simulink library "xblocks_library_pfbs"  (Simulink 7.6)
settings: Solver=ode45  SolverMode=SingleTasking  StartTime=0.0  StopTime=10.0  RelTol=1e-3
libraries: xbsIndex_r4 x369, monroe_library x47
(part 1 of 7)
settings Model: Creator=mdexter  LastModifiedBy=ptcs

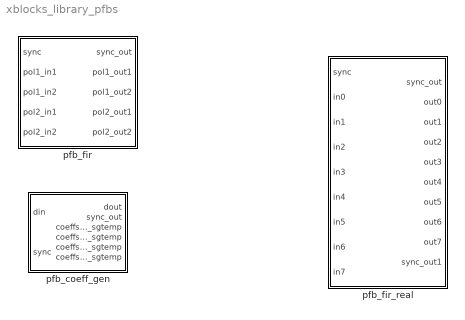
== system xblocks_library_pfbs ==
  pfb_coeff_gen : Subsystem  mask(pfb_coeff_gen){PFBSize=6, CoeffBitWidth=8, TotalTaps=4, CoeffDistMem=0, WindowType=hamming, bram_latency=2, n_inputs=0, nput=0, fwidth=1}
      mask prompts: PFBSize "Size of PFB: (2^? pnts)"; CoeffBitWidth "Bitwidth of Coefficients:"; TotalTaps "Total Number of Taps:"; CoeffDistMem "Implement Coeff Gen in Distributed Memory"; WindowType "Windowing Function:"; bram_latency "BRAM Latency"; n_inputs "Number of Simultaneous Inputs: (2^?)"; nput "This is input number:"; fwidth "Bin Width (normal=1)"
      mask init:
      | config.source = str2func('pfb_coeff_gen_init_xblock');
      | config.toplevel = gcb;
      | config.depend = get_dependlist('pfb_coeff_gen');
      | set_param(gcb,'LinkStatus','inactive');
      | xBlock(config, {config.toplevel, ...
      |     PFBSize, ...
      |     CoeffBitWidth, ...
      |     TotalTaps, ...
      |     CoeffDistMem, ...
      |     WindowType, ...
      |     bram_latency, ...
      |     n_inputs, ...
      |     nput, ...
      |     fwidth});
      settings: AttributesFormatString=PFBSize=6, n_inputs=0, taps=4
  pfb_fir : Subsystem  mask(pfb_fir){PFBSize=5, TotalTaps=2, WindowType=hamming, n_inputs=1, MakeBiplex=on, BitWidthIn=8, BitWidthOut=18, CoeffBitWidth=18, CoeffDistMem=off, add_latency=1, mult_latency=2, bram_latency=2, quantization=Round  (unbiased: +/- Inf), fwidth=1, oversample_factor=1, oversample_index=0, specify_mult=off, mult_spec=[2                                      2]}
      mask prompts: PFBSize "Size of PFB: (2^? pnts)"; TotalTaps "Total Number of Taps:"; WindowType "Windowing Function:"; n_inputs "Number of Simultaneous Inputs: (2^?)"; MakeBiplex "Make Biplex"; BitWidthIn "Input Bitwidth:"; BitWidthOut "Output Bitwidth:"; CoeffBitWidth "Coefficient Bitwidth:"; CoeffDistMem "Use Distributed Memory for Coeffs"; add_latency "Add Latency"; mult_latency "Mult Latency"; bram_latency "BRAM Latency"; quantization "Quantization Behavior"; fwidth "Bin Width Scaling (normal=1)"; oversample_factor "Oversampling factor"; oversample_index "Oversampling index"; specify_mult "Specify multiplier use (behavioral if not specified)"; mult_spec "Multiplier specification (0=core, 1=embedded, 2=behavioural) (left=1st tap)"
      mask init:
      | config.source = str2func('pfb_fir_init_xblock');
      | config.toplevel = gcb;
      | config.depend = get_dependlist('pfb_fir');
      | set_param(gcb,'LinkStatus','inactive');
      | xBlock(config,{config.toplevel, ...
      |     'PFBSize', PFBSize, ...
      |     'TotalTaps', TotalTaps, ...
      |     'WindowType', WindowType, ...
      |     'n_inputs', n_inputs, ...
      |     'MakeBiplex', MakeBiplex, ...
      |     'BitWidthIn', BitWidthIn, ...
      |     'BitWidthOut', BitWidthOut, ...
      |     'CoeffBitWidth', CoeffBitWidth, ...
      |     'CoeffDistMem', CoeffDistMem, ...
      |     'add_latency', add_latency, ...
      |     'mult_latency', mult_latency, ...
      |     'bram_latency', bram_latency, ...
      |     'quantization', quantization, ...
      |     'fwidth', fwidth,...
      |     'oversample_factor', oversample_factor,...
      |     'oversample_index', oversample_index,...
      |     'specify_mult', specify_mult,...
      |     'mult_spec', mult_spec});
      settings: AttributesFormatString=taps=2, add_latency=1
      mask Help: eval('xlWeb(''http://casper.berkeley.edu/wiki/Pfb_fir'')')
      mask StyleString: edit,edit,popup(bartlett|barthannwin|blackman|blackmanharris|bohamwin|chebwin|flattopwin|gausswin|hamming|hann|kaiser|nuttallwin|parzenwin|rectwin|tukeywin|triang|userwindow),edit,checkbox,edit,edit,edit,checkbox,edit,edit,edit,popup(Truncate|Round  (unbiased: +/- Inf)|Round  (unbiased: Even Values)),edit,edit,edit,checkbox,edit
      mask CallbackString:
      | |%num_taps = eval(get_param(gcb, 'TotalTaps'));
      | %old_vec = eval(get_param(gcb, 'mult_spec'));
      | 
      | %vec = 2.*ones(1,num_taps);
      | %old_size = length(old_vec);
      | 
      | %if(old_size <= num_taps),
      | %   new_size = old_size;
      | %else,
      | %    new_size = num_taps;
      | %end
      | 
      | %for n = 1:new_size, vec(n) = old_vec(n); end
      | %set_param(gcb, 'mult_spec', mat2str(vec));||||||||||||%num_taps = eval(get_param(gcb, 'TotalTaps'));
      | %old_vec = eval(get_param(gcb, 'mult_spec'));
      | 
      | %vec = 2.*ones(1,num_taps);
      | %old_size = length(old_vec);
      | 
      | %if(old_size <= num_taps),
      | %    new_size = old_size;
      | %else,
      | %    new_size = num_taps;
      | %end
      | 
      | %for n = 1:new_size, vec(n) = old_vec(n); end
      | %set_param(gcb, 'mult_spec', mat2str(vec));|||%specify_mult = get_param(gcb,'specify_mult');
      | %if( strcmp(specify_mult,'off')),
      | %    set_param(gcb, 'MaskEnables', {'on','on','on','on','on','on','on','on','on','on','on','on','on','on','on','off'});
      | %else
      | %    set_param(gcb, 'MaskEnables', {'on','on','on','on','on','on','on','on','on','on','on','on','on','on','on','on'});
      | %end
      | 
      | |%specify_mult = get_param(gcb,'specify_mult');
      | %if( strcmp(specify_mult,'off')),
      | %    set_param(gcb, 'MaskEnables', {'on','on','on','on','on','on','on','on','on','on','on','on','on','on','on','off'});
      | %else
      | %    set_param(gcb, 'MaskEnables', {'on','on','on','on','on','on','on','on','on','on','on','on','on','on','on','on'});
      | %end
  pfb_fir_real : Subsystem  mask(pfb_coeff_gen_dual){pfb_size=14, n_sim_inputs=3, n_taps=4, data_n_bits=18, coeff_n_bits=18, output_bit_width=18, window_fn=hamming, bin_width=1, end_scale_val=1, endDelay=off, cheap_sync=off, autoplace_mode='Attached to ADC0', autoplace_optimize=off, bram_latency_coeff=off, bram_latency_delay=off, register_counter=off, pack_delays=on}
      mask prompts: pfb_size "PFB Size (2^?)"; n_sim_inputs "# Simultaneous Inputs (2^?); Max=6"; n_taps "# Taps"; data_n_bits "Input bit Width"; coeff_n_bits "# Coefficient Bits"; output_bit_width "Output bit width"; window_fn "Window Function"; bin_width "Channel Width"; end_scale_val "Downscale at end (2^?)"; endDelay "Delay at end?"; cheap_sync "Use cheap Sync hardware?"; autoplace_mode "Autoplacement Mode?"; autoplace_optimize "Optimize parameters for auto-placement? (settings below here ignored)"; bram_latency_coeff "Register Coefficient Brams?"; bram_latency_delay "Register Delay Brams?"; register_counter "Register Delay Counters? (0 or 1)"; pack_delays "Pack delays cross-input?"
      mask init:
      | global drawing_parameters;
      | % drawing_parameters.pfb_size=pfb_size;
      | % drawing_parameters.n_sim_inputs=n_sim_inputs;
      | % drawing_parameters.n_taps=n_taps;
      | % drawing_parameters.data_n_bits=data_n_bits;
      | % drawing_parameters.data_bin_pt=data_bin_pt;
      | % drawing_parameters.coeff_n_bits=coeff_n_bits;
      | % drawing_parameters.coeff_bin_pt=coeff_n_bits-1;
      | % drawing_parameters.window_fn=window_fn;
      | % drawing_parameters.mem_type=mem_type;
      | % drawing_parameters.bram_latency=bram_latency;
      | % drawing_parameters.bin_width=bin_width;
      | % drawing_parameters.end_scale_val=end_scale_val;
      | % drawing_parameters.cheap_sync=cheap_sync;
      | config.source=str2func('pfb_improved_draw');
      | config.toplevel=gcb;
      | config.debug=0;
      | config.depend={'pfb_improved_draw.m','pfb_coeff_gen_dual_draw.m'};
      | xBlock(config,{pfb_size,n_sim_inputs,n_taps,data_n_bits,coeff_n_bits, ...
      |                output_bit_width,window_fn,bram_latency_coeff+2,bram_latency_delay+2,bin_width,end_scale_val,endDelay, cheap_sync,register_counter, pack_delays, autoplace_mode, autoplace_optimize});
      mask StyleString: edit,edit,edit,edit,edit,edit,popup(bartlett|barthannwin|blackman|blackmanharris|bohamwin|chebwin|flattopwin|gausswin|hamming|hann|kaiser|nuttallwin|parzenwin|rectwin|tukeywin|triang),edit,edit,checkbox,checkbox,popup('Attached to ADC0'|'Attached to ADC1'|'Attached to both ADC0 and ADC1 (interleaved)'),checkbox,checkbox,checkbox,checkbox,checkbox

== system xblocks_library_pfbs/pfb_coeff_gen ==
  din : Inport
  sync : Inport  Port=2
  Counter : xbsIndex_r4/Counter  cnt_type=Free Running  cnt_to=Inf  operation=Up  start_count=0  cnt_by_val=1  arith_type=Unsigned  n_bits=6  bin_pt=0  load_pin=off  rst=on  en=off  explicit_period=on  period=1  dbl_ovrd=off  use_behavioral_HDL=off  implementation=Fabric  use_rpm=on  block_type=counter
  Delay : xbsIndex_r4/Delay  rst=off  infoeditControl=Selection of Reset will increase slice count due to use of real FFs and instead of SRLs  en=off  latency=3  dbl_ovrd=off  reg_retiming=off  block_type=delay
  Delay1 : xbsIndex_r4/Delay  rst=off  infoeditControl=Selection of Reset will increase slice count due to use of real FFs and instead of SRLs  en=off  latency=3  dbl_ovrd=off  reg_retiming=off  block_type=delay
  dout : Outport
  sync_out : Outport  Port=2
  coeffs1_sgtemp : Outport  Port=3
  coeffs2_sgtemp : Outport  Port=4
  coeffs3_sgtemp : Outport  Port=5
  coeffs4_sgtemp : Outport  Port=6
  wires:
  sync/1 -> Counter/1, Delay/1
  Delay/1 -> sync_out/1
  din/1 -> Delay1/1
  Delay1/1 -> dout/1

== system xblocks_library_pfbs/pfb_fir ==
  sync : Inport
  pol1_in1 : Inport  Port=2
  pol1_in2 : Inport  Port=3
  pol2_in1 : Inport  Port=4
  pol2_in2 : Inport  Port=5
  pfb_row_11 : Subsystem
  pfb_row_12 : Subsystem
  pfb_row_21 : Subsystem
  pfb_row_22 : Subsystem
  sync_out : Outport
  pol1_out1 : Outport  Port=2
  pol1_out2 : Outport  Port=3
  pol2_out1 : Outport  Port=4
  pol2_out2 : Outport  Port=5
  wires:
  sync/1 -> pfb_row_22/2(sync), pfb_row_21/2(sync), pfb_row_12/2(sync), pfb_row_11/2(sync)
  pfb_row_22/2(out) -> pol2_out2/1
  pol2_in2/1 -> pfb_row_22/1(din)
  pfb_row_21/2(out) -> pol2_out1/1
  pol2_in1/1 -> pfb_row_21/1(din)
  pfb_row_12/2(out) -> pol1_out2/1
  pol1_in2/1 -> pfb_row_12/1(din)
  pfb_row_11/2(out) -> pol1_out1/1
  pfb_row_11/1(sync_out) -> sync_out/1
  pol1_in1/1 -> pfb_row_11/1(din)

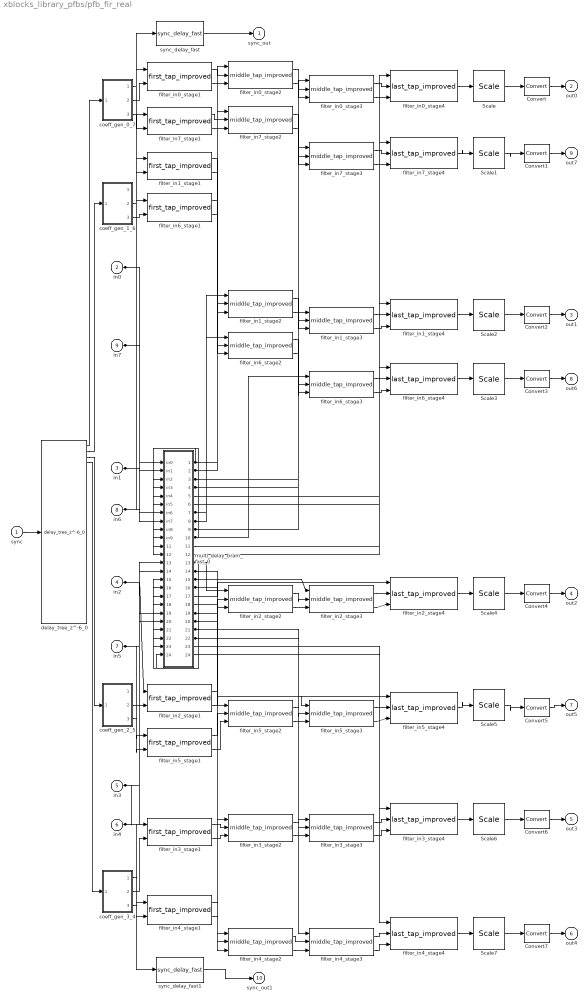
== system xblocks_library_pfbs/pfb_fir_real ==
  sync : Inport
  in0 : Inport  Port=2
  in1 : Inport  Port=3
  in2 : Inport  Port=4
  in3 : Inport  Port=5
  in4 : Inport  Port=6
  in5 : Inport  Port=7
  in6 : Inport  Port=8
  in7 : Inport  Port=9
  Convert{,1..7} (8 alike) : xbsIndex_r4/Convert  gui_display_data_type=Fixed-point  arith_type="Signed  (2's comp)"  n_bits=18  bin_pt=17  float_type=Single  exp_bits=8  fraction_bits=24  quantization=Truncate  overflow=Wrap  en=off  latency=0  dbl_ovrd=off  pipeline=off  block_type=convert
  Scale{,1..7} (8 alike) : xbsIndex_r4/Scale  scale_factor=-1  dbl_ovrd=off  block_type=scale
  coeff_gen_0_7 : Subsystem
  coeff_gen_1_6 : Subsystem
  coeff_gen_2_5 : Subsystem
  coeff_gen_3_4 : Subsystem
  delay_tree_z^-6_0 : monroe_library/delay_tree_z^-6_0  SystemSampleTime=-1
  filter_in0_stage1 : monroe_library/first_tap_improved  SystemSampleTime=-1  data_bin_pt=17  coeff_bit_width=18
  filter_in0_stage2 : monroe_library/middle_tap_improved  SystemSampleTime=-1  data_bin_pt=17  coeff_bit_width=18  stage_num=2
  filter_in0_stage3 : monroe_library/middle_tap_improved  SystemSampleTime=-1  data_bin_pt=17  coeff_bit_width=18  stage_num=3
  filter_in0_stage4 : monroe_library/last_tap_improved  SystemSampleTime=-1  data_bin_pt=17  coeff_bin_pt=17  stage_num=4
  filter_in1_stage1 : monroe_library/first_tap_improved  SystemSampleTime=-1  data_bin_pt=17  coeff_bit_width=18
  filter_in1_stage2 : monroe_library/middle_tap_improved  SystemSampleTime=-1  data_bin_pt=17  coeff_bit_width=18  stage_num=2
  filter_in1_stage3 : monroe_library/middle_tap_improved  SystemSampleTime=-1  data_bin_pt=17  coeff_bit_width=18  stage_num=3
  filter_in1_stage4 : monroe_library/last_tap_improved  SystemSampleTime=-1  data_bin_pt=17  coeff_bin_pt=17  stage_num=4
  filter_in2_stage1 : monroe_library/first_tap_improved  SystemSampleTime=-1  data_bin_pt=17  coeff_bit_width=18
  filter_in2_stage2 : monroe_library/middle_tap_improved  SystemSampleTime=-1  data_bin_pt=17  coeff_bit_width=18  stage_num=2
  filter_in2_stage3 : monroe_library/middle_tap_improved  SystemSampleTime=-1  data_bin_pt=17  coeff_bit_width=18  stage_num=3
  filter_in2_stage4 : monroe_library/last_tap_improved  SystemSampleTime=-1  data_bin_pt=17  coeff_bin_pt=17  stage_num=4
  filter_in3_stage1 : monroe_library/first_tap_improved  SystemSampleTime=-1  data_bin_pt=17  coeff_bit_width=18
  filter_in3_stage2 : monroe_library/middle_tap_improved  SystemSampleTime=-1  data_bin_pt=17  coeff_bit_width=18  stage_num=2
  filter_in3_stage3 : monroe_library/middle_tap_improved  SystemSampleTime=-1  data_bin_pt=17  coeff_bit_width=18  stage_num=3
  filter_in3_stage4 : monroe_library/last_tap_improved  SystemSampleTime=-1  data_bin_pt=17  coeff_bin_pt=17  stage_num=4
  filter_in4_stage1 : monroe_library/first_tap_improved  SystemSampleTime=-1  data_bin_pt=17  coeff_bit_width=18
  filter_in4_stage2 : monroe_library/middle_tap_improved  SystemSampleTime=-1  data_bin_pt=17  coeff_bit_width=18  stage_num=2
  filter_in4_stage3 : monroe_library/middle_tap_improved  SystemSampleTime=-1  data_bin_pt=17  coeff_bit_width=18  stage_num=3
  filter_in4_stage4 : monroe_library/last_tap_improved  SystemSampleTime=-1  data_bin_pt=17  coeff_bin_pt=17  stage_num=4
  filter_in5_stage1 : monroe_library/first_tap_improved  SystemSampleTime=-1  data_bin_pt=17  coeff_bit_width=18
  filter_in5_stage2 : monroe_library/middle_tap_improved  SystemSampleTime=-1  data_bin_pt=17  coeff_bit_width=18  stage_num=2
  filter_in5_stage3 : monroe_library/middle_tap_improved  SystemSampleTime=-1  data_bin_pt=17  coeff_bit_width=18  stage_num=3
  filter_in5_stage4 : monroe_library/last_tap_improved  SystemSampleTime=-1  data_bin_pt=17  coeff_bin_pt=17  stage_num=4
  filter_in6_stage1 : monroe_library/first_tap_improved  SystemSampleTime=-1  data_bin_pt=17  coeff_bit_width=18
  filter_in6_stage2 : monroe_library/middle_tap_improved  SystemSampleTime=-1  data_bin_pt=17  coeff_bit_width=18  stage_num=2
  filter_in6_stage3 : monroe_library/middle_tap_improved  SystemSampleTime=-1  data_bin_pt=17  coeff_bit_width=18  stage_num=3
  filter_in6_stage4 : monroe_library/last_tap_improved  SystemSampleTime=-1  data_bin_pt=17  coeff_bin_pt=17  stage_num=4
  filter_in7_stage1 : monroe_library/first_tap_improved  SystemSampleTime=-1  data_bin_pt=17  coeff_bit_width=18
  filter_in7_stage2 : monroe_library/middle_tap_improved  SystemSampleTime=-1  data_bin_pt=17  coeff_bit_width=18  stage_num=2
  filter_in7_stage3 : monroe_library/middle_tap_improved  SystemSampleTime=-1  data_bin_pt=17  coeff_bit_width=18  stage_num=3
  filter_in7_stage4 : monroe_library/last_tap_improved  SystemSampleTime=-1  data_bin_pt=17  coeff_bin_pt=17  stage_num=4
  multi_delay_bram_fast_0 : Subsystem
  sync_delay_fast : monroe_library/sync_delay_fast  SystemSampleTime=-1  delay_len=6142
  sync_delay_fast1 : monroe_library/sync_delay_fast  SystemSampleTime=-1  delay_len=6142
  sync_out : Outport
  out0 : Outport  Port=2
  out1 : Outport  Port=3
  out2 : Outport  Port=4
  out3 : Outport  Port=5
  out4 : Outport  Port=6
  out5 : Outport  Port=7
  out6 : Outport  Port=8
  out7 : Outport  Port=9
  sync_out1 : Outport  Port=10
  wires:
  in0/1 -> multi_delay_bram_fast_0/1(in0), filter_in0_stage1/1
  in7/1 -> multi_delay_bram_fast_0/2(in1), filter_in7_stage1/1
  in1/1 -> filter_in1_stage1/1, multi_delay_bram_fast_0/7(in6)
  in6/1 -> filter_in6_stage1/1, multi_delay_bram_fast_0/8(in7)
  in2/1 -> filter_in2_stage1/1, multi_delay_bram_fast_0/13(in12)
  in5/1 -> filter_in5_stage1/1, multi_delay_bram_fast_0/14(in13)
  in3/1 -> filter_in3_stage1/1, multi_delay_bram_fast_0/19(in18)
  in4/1 -> filter_in4_stage1/1, multi_delay_bram_fast_0/20(in19)
  multi_delay_bram_fast_0/1(out0) -> filter_in0_stage2/1, multi_delay_bram_fast_0/3(in2)
  multi_delay_bram_fast_0/2(out1) -> filter_in7_stage2/1, multi_delay_bram_fast_0/4(in3)
  multi_delay_bram_fast_0/3(out2) -> filter_in0_stage3/1, multi_delay_bram_fast_0/5(in4)
  multi_delay_bram_fast_0/4(out3) -> filter_in7_stage3/1, multi_delay_bram_fast_0/6(in5)
  multi_delay_bram_fast_0/7(out6) -> filter_in1_stage2/1, multi_delay_bram_fast_0/9(in8)
  multi_delay_bram_fast_0/8(out7) -> filter_in6_stage2/1, multi_delay_bram_fast_0/10(in9)
  multi_delay_bram_fast_0/9(out8) -> filter_in1_stage3/1, multi_delay_bram_fast_0/11(in10)
  multi_delay_bram_fast_0/10(out9) -> filter_in6_stage3/1, multi_delay_bram_fast_0/12(in11)
  multi_delay_bram_fast_0/13(out12) -> filter_in2_stage2/1, multi_delay_bram_fast_0/15(in14)
  multi_delay_bram_fast_0/14(out13) -> filter_in5_stage2/1, multi_delay_bram_fast_0/16(in15)
  multi_delay_bram_fast_0/15(out14) -> filter_in2_stage3/1, multi_delay_bram_fast_0/17(in16)
  multi_delay_bram_fast_0/16(out15) -> filter_in5_stage3/1, multi_delay_bram_fast_0/18(in17)
  multi_delay_bram_fast_0/19(out18) -> filter_in3_stage2/1, multi_delay_bram_fast_0/21(in20)
  multi_delay_bram_fast_0/20(out19) -> filter_in4_stage2/1, multi_delay_bram_fast_0/22(in21)
  multi_delay_bram_fast_0/21(out20) -> filter_in3_stage3/1, multi_delay_bram_fast_0/23(in22)
  multi_delay_bram_fast_0/22(out21) -> filter_in4_stage3/1, multi_delay_bram_fast_0/24(in23)
  sync_delay_fast1/1 -> sync_out1/1
  coeff_gen_3_4/1(sync_out) -> sync_delay_fast1/1
  sync_delay_fast/1 -> sync_out/1
  coeff_gen_0_7/1(sync_out) -> sync_delay_fast/1
  Convert7/1 -> out4/1
  Scale7/1 -> Convert7/1
  Convert6/1 -> out3/1
  Scale6/1 -> Convert6/1
  filter_in4_stage4/1 -> Scale7/1
  filter_in3_stage4/1 -> Scale6/1
  filter_in4_stage3/2 -> filter_in4_stage4/3
  filter_in4_stage3/1 -> filter_in4_stage4/2
  multi_delay_bram_fast_0/24(out23) -> filter_in4_stage4/1
  filter_in3_stage3/2 -> filter_in3_stage4/3
  filter_in3_stage3/1 -> filter_in3_stage4/2
  multi_delay_bram_fast_0/23(out22) -> filter_in3_stage4/1
  filter_in4_stage2/2 -> filter_in4_stage3/3
  filter_in4_stage2/1 -> filter_in4_stage3/2
  filter_in3_stage2/2 -> filter_in3_stage3/3
  filter_in3_stage2/1 -> filter_in3_stage3/2
  filter_in4_stage1/2 -> filter_in4_stage2/3
  filter_in4_stage1/1 -> filter_in4_stage2/2
  filter_in3_stage1/2 -> filter_in3_stage2/3
  filter_in3_stage1/1 -> filter_in3_stage2/2
  coeff_gen_3_4/3(coeff_rev) -> filter_in4_stage1/2
  coeff_gen_3_4/2(coeff) -> filter_in3_stage1/2
  delay_tree_z^-6_0/4 -> coeff_gen_3_4/1(sync)
  Convert5/1 -> out5/1
  Scale5/1 -> Convert5/1
  Convert4/1 -> out2/1
  Scale4/1 -> Convert4/1
  filter_in5_stage4/1 -> Scale5/1
  filter_in2_stage4/1 -> Scale4/1
  filter_in5_stage3/2 -> filter_in5_stage4/3
  filter_in5_stage3/1 -> filter_in5_stage4/2
  multi_delay_bram_fast_0/18(out17) -> filter_in5_stage4/1
  filter_in2_stage3/2 -> filter_in2_stage4/3
  filter_in2_stage3/1 -> filter_in2_stage4/2
  multi_delay_bram_fast_0/17(out16) -> filter_in2_stage4/1
  filter_in5_stage2/2 -> filter_in5_stage3/3
  filter_in5_stage2/1 -> filter_in5_stage3/2
  filter_in2_stage2/2 -> filter_in2_stage3/3
  filter_in2_stage2/1 -> filter_in2_stage3/2
  filter_in5_stage1/2 -> filter_in5_stage2/3
  filter_in5_stage1/1 -> filter_in5_stage2/2
  filter_in2_stage1/2 -> filter_in2_stage2/3
  filter_in2_stage1/1 -> filter_in2_stage2/2
  coeff_gen_2_5/3(coeff_rev) -> filter_in5_stage1/2
  coeff_gen_2_5/2(coeff) -> filter_in2_stage1/2
  delay_tree_z^-6_0/3 -> coeff_gen_2_5/1(sync)
  Convert3/1 -> out6/1
  Scale3/1 -> Convert3/1
  Convert2/1 -> out1/1
  Scale2/1 -> Convert2/1
  filter_in6_stage4/1 -> Scale3/1
  filter_in1_stage4/1 -> Scale2/1
  filter_in6_stage3/2 -> filter_in6_stage4/3
  filter_in6_stage3/1 -> filter_in6_stage4/2
  multi_delay_bram_fast_0/12(out11) -> filter_in6_stage4/1
  filter_in1_stage3/2 -> filter_in1_stage4/3
  filter_in1_stage3/1 -> filter_in1_stage4/2
  multi_delay_bram_fast_0/11(out10) -> filter_in1_stage4/1
  filter_in6_stage2/2 -> filter_in6_stage3/3
  filter_in6_stage2/1 -> filter_in6_stage3/2
  filter_in1_stage2/2 -> filter_in1_stage3/3
  filter_in1_stage2/1 -> filter_in1_stage3/2
  filter_in6_stage1/2 -> filter_in6_stage2/3
  filter_in6_stage1/1 -> filter_in6_stage2/2
  filter_in1_stage1/2 -> filter_in1_stage2/3
  filter_in1_stage1/1 -> filter_in1_stage2/2
  coeff_gen_1_6/3(coeff_rev) -> filter_in6_stage1/2
  coeff_gen_1_6/2(coeff) -> filter_in1_stage1/2
  delay_tree_z^-6_0/2 -> coeff_gen_1_6/1(sync)
  Convert1/1 -> out7/1
  Scale1/1 -> Convert1/1
  Convert/1 -> out0/1
  Scale/1 -> Convert/1
  filter_in7_stage4/1 -> Scale1/1
  filter_in0_stage4/1 -> Scale/1
  filter_in7_stage3/2 -> filter_in7_stage4/3
  filter_in7_stage3/1 -> filter_in7_stage4/2
  multi_delay_bram_fast_0/6(out5) -> filter_in7_stage4/1
  filter_in0_stage3/2 -> filter_in0_stage4/3
  filter_in0_stage3/1 -> filter_in0_stage4/2
  multi_delay_bram_fast_0/5(out4) -> filter_in0_stage4/1
  filter_in7_stage2/2 -> filter_in7_stage3/3
  filter_in7_stage2/1 -> filter_in7_stage3/2
  filter_in0_stage2/2 -> filter_in0_stage3/3
  filter_in0_stage2/1 -> filter_in0_stage3/2
  filter_in7_stage1/2 -> filter_in7_stage2/3
  filter_in7_stage1/1 -> filter_in7_stage2/2
  filter_in0_stage1/2 -> filter_in0_stage2/3
  filter_in0_stage1/1 -> filter_in0_stage2/2
  coeff_gen_0_7/3(coeff_rev) -> filter_in7_stage1/2
  coeff_gen_0_7/2(coeff) -> filter_in0_stage1/2
  delay_tree_z^-6_0/1 -> coeff_gen_0_7/1(sync)
  sync/1 -> delay_tree_z^-6_0/1

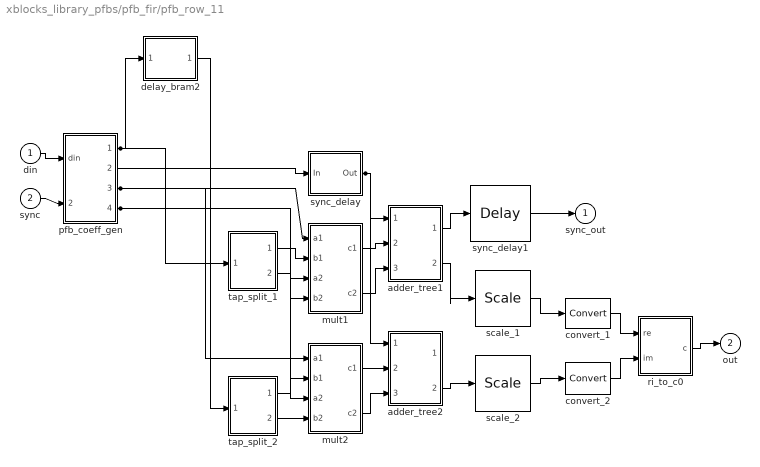
== system xblocks_library_pfbs/pfb_fir/pfb_row_11 ==
  din : Inport
  sync : Inport  Port=2
  adder_tree1 : Subsystem
  adder_tree2 : Subsystem
  convert_1 : xbsIndex_r4/Convert  gui_display_data_type=Fixed-point  arith_type="Signed  (2's comp)"  n_bits=18  bin_pt=17  float_type=Single  exp_bits=8  fraction_bits=24  quantization="Round  (unbiased: +/- Inf)"  overflow=Saturate  en=off  latency=2  dbl_ovrd=off  pipeline=on  block_type=convert
  convert_2 : xbsIndex_r4/Convert  gui_display_data_type=Fixed-point  arith_type="Signed  (2's comp)"  n_bits=18  bin_pt=17  float_type=Single  exp_bits=8  fraction_bits=24  quantization="Round  (unbiased: +/- Inf)"  overflow=Saturate  en=off  latency=2  dbl_ovrd=off  pipeline=on  block_type=convert
  delay_bram2 : Subsystem
  mult1 : Subsystem
  mult2 : Subsystem
  pfb_coeff_gen : Subsystem
      settings: AttributesFormatString=PFBSize=5, n_inputs=1, taps=2
  ri_to_c0 : Subsystem
  scale_1 : xbsIndex_r4/Scale  scale_factor=-2  dbl_ovrd=off  block_type=scale
  scale_2 : xbsIndex_r4/Scale  scale_factor=-2  dbl_ovrd=off  block_type=scale
  sync_delay : Subsystem
  sync_delay1 : xbsIndex_r4/Delay  rst=off  infoeditControl=Selection of Reset will increase slice count due to use of real FFs and instead of SRLs  en=off  latency=2  dbl_ovrd=off  reg_retiming=off  block_type=delay
  tap_split_1 : Subsystem
      settings: AttributesFormatString=Fix_8_7
  tap_split_2 : Subsystem
      settings: AttributesFormatString=Fix_8_7
  sync_out : Outport
  out : Outport  Port=2
  wires:
  pfb_coeff_gen/1(dout) -> tap_split_1/1(inport), delay_bram2/1(din_1_1)
  pfb_coeff_gen/3(coeffs1) -> mult2/1(a1), mult1/1(a1)
  pfb_coeff_gen/4(coeffs2) -> mult2/3(a2), mult1/3(a2)
  sync_delay/1(Out) -> adder_tree2/1(sync), adder_tree1/1(sync)
  ri_to_c0/1(c) -> out/1
  convert_2/1 -> ri_to_c0/2(im)
  convert_1/1 -> ri_to_c0/1(re)
  scale_2/1 -> convert_2/1
  adder_tree2/2(dout) -> scale_2/1
  mult2/2(c2) -> adder_tree2/3(din_2)
  mult2/1(c1) -> adder_tree2/2(din_1)
  tap_split_2/2(outport2) -> mult2/4(b2)
  tap_split_1/2(outport2) -> mult2/2(b1)
  sync_delay1/1 -> sync_out/1
  adder_tree1/1(sync_out) -> sync_delay1/1
  scale_1/1 -> convert_1/1
  adder_tree1/2(dout) -> scale_1/1
  mult1/2(c2) -> adder_tree1/3(din_2)
  mult1/1(c1) -> adder_tree1/2(din_1)
  tap_split_2/1(outport1) -> mult1/4(b2)
  tap_split_1/1(outport1) -> mult1/2(b1)
  delay_bram2/1(dout_1_1) -> tap_split_2/1(inport)
  pfb_coeff_gen/2(sync_out) -> sync_delay/1(In)
  sync/1 -> pfb_coeff_gen/2(sync)
  din/1 -> pfb_coeff_gen/1(din)

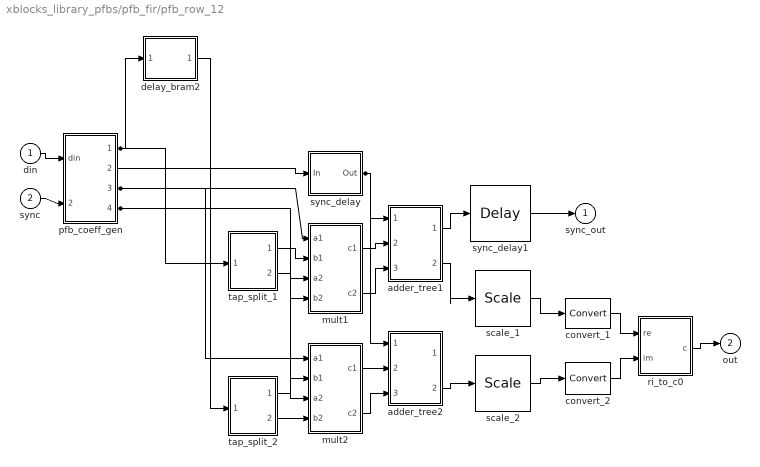
== system xblocks_library_pfbs/pfb_fir/pfb_row_12 ==
  din : Inport
  sync : Inport  Port=2
  adder_tree1 : Subsystem
  adder_tree2 : Subsystem
  convert_1 : xbsIndex_r4/Convert  gui_display_data_type=Fixed-point  arith_type="Signed  (2's comp)"  n_bits=18  bin_pt=17  float_type=Single  exp_bits=8  fraction_bits=24  quantization="Round  (unbiased: +/- Inf)"  overflow=Saturate  en=off  latency=2  dbl_ovrd=off  pipeline=on  block_type=convert
  convert_2 : xbsIndex_r4/Convert  gui_display_data_type=Fixed-point  arith_type="Signed  (2's comp)"  n_bits=18  bin_pt=17  float_type=Single  exp_bits=8  fraction_bits=24  quantization="Round  (unbiased: +/- Inf)"  overflow=Saturate  en=off  latency=2  dbl_ovrd=off  pipeline=on  block_type=convert
  delay_bram2 : Subsystem
  mult1 : Subsystem
  mult2 : Subsystem
  pfb_coeff_gen : Subsystem
      settings: AttributesFormatString=PFBSize=5, n_inputs=1, taps=2
  ri_to_c0 : Subsystem
  scale_1 : xbsIndex_r4/Scale  scale_factor=-2  dbl_ovrd=off  block_type=scale
  scale_2 : xbsIndex_r4/Scale  scale_factor=-2  dbl_ovrd=off  block_type=scale
  sync_delay : Subsystem
  sync_delay1 : xbsIndex_r4/Delay  rst=off  infoeditControl=Selection of Reset will increase slice count due to use of real FFs and instead of SRLs  en=off  latency=2  dbl_ovrd=off  reg_retiming=off  block_type=delay
  tap_split_1 : Subsystem
      settings: AttributesFormatString=Fix_8_7
  tap_split_2 : Subsystem
      settings: AttributesFormatString=Fix_8_7
  sync_out : Outport
  out : Outport  Port=2
  wires:
  pfb_coeff_gen/1(dout) -> tap_split_1/1(inport), delay_bram2/1(din_1_1)
  pfb_coeff_gen/3(coeffs1) -> mult2/1(a1), mult1/1(a1)
  pfb_coeff_gen/4(coeffs2) -> mult2/3(a2), mult1/3(a2)
  sync_delay/1(Out) -> adder_tree2/1(sync), adder_tree1/1(sync)
  ri_to_c0/1(c) -> out/1
  convert_2/1 -> ri_to_c0/2(im)
  convert_1/1 -> ri_to_c0/1(re)
  scale_2/1 -> convert_2/1
  adder_tree2/2(dout) -> scale_2/1
  mult2/2(c2) -> adder_tree2/3(din_2)
  mult2/1(c1) -> adder_tree2/2(din_1)
  tap_split_2/2(outport2) -> mult2/4(b2)
  tap_split_1/2(outport2) -> mult2/2(b1)
  sync_delay1/1 -> sync_out/1
  adder_tree1/1(sync_out) -> sync_delay1/1
  scale_1/1 -> convert_1/1
  adder_tree1/2(dout) -> scale_1/1
  mult1/2(c2) -> adder_tree1/3(din_2)
  mult1/1(c1) -> adder_tree1/2(din_1)
  tap_split_2/1(outport1) -> mult1/4(b2)
  tap_split_1/1(outport1) -> mult1/2(b1)
  delay_bram2/1(dout_1_1) -> tap_split_2/1(inport)
  pfb_coeff_gen/2(sync_out) -> sync_delay/1(In)
  sync/1 -> pfb_coeff_gen/2(sync)
  din/1 -> pfb_coeff_gen/1(din)

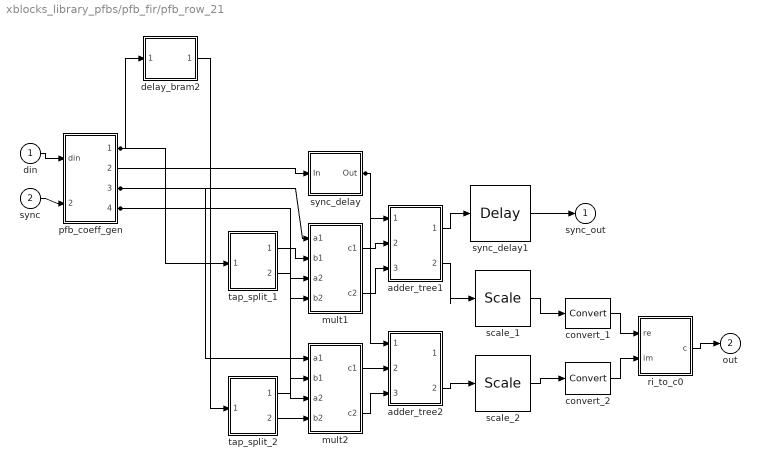
== system xblocks_library_pfbs/pfb_fir/pfb_row_21 ==
  din : Inport
  sync : Inport  Port=2
  adder_tree1 : Subsystem
  adder_tree2 : Subsystem
  convert_1 : xbsIndex_r4/Convert  gui_display_data_type=Fixed-point  arith_type="Signed  (2's comp)"  n_bits=18  bin_pt=17  float_type=Single  exp_bits=8  fraction_bits=24  quantization="Round  (unbiased: +/- Inf)"  overflow=Saturate  en=off  latency=2  dbl_ovrd=off  pipeline=on  block_type=convert
  convert_2 : xbsIndex_r4/Convert  gui_display_data_type=Fixed-point  arith_type="Signed  (2's comp)"  n_bits=18  bin_pt=17  float_type=Single  exp_bits=8  fraction_bits=24  quantization="Round  (unbiased: +/- Inf)"  overflow=Saturate  en=off  latency=2  dbl_ovrd=off  pipeline=on  block_type=convert
  delay_bram2 : Subsystem
  mult1 : Subsystem
  mult2 : Subsystem
  pfb_coeff_gen : Subsystem
      settings: AttributesFormatString=PFBSize=5, n_inputs=1, taps=2
  ri_to_c0 : Subsystem
  scale_1 : xbsIndex_r4/Scale  scale_factor=-2  dbl_ovrd=off  block_type=scale
  scale_2 : xbsIndex_r4/Scale  scale_factor=-2  dbl_ovrd=off  block_type=scale
  sync_delay : Subsystem
  sync_delay1 : xbsIndex_r4/Delay  rst=off  infoeditControl=Selection of Reset will increase slice count due to use of real FFs and instead of SRLs  en=off  latency=2  dbl_ovrd=off  reg_retiming=off  block_type=delay
  tap_split_1 : Subsystem
      settings: AttributesFormatString=Fix_8_7
  tap_split_2 : Subsystem
      settings: AttributesFormatString=Fix_8_7
  sync_out : Outport
  out : Outport  Port=2
  wires:
  pfb_coeff_gen/1(dout) -> tap_split_1/1(inport), delay_bram2/1(din_1_1)
  pfb_coeff_gen/3(coeffs1) -> mult2/1(a1), mult1/1(a1)
  pfb_coeff_gen/4(coeffs2) -> mult2/3(a2), mult1/3(a2)
  sync_delay/1(Out) -> adder_tree2/1(sync), adder_tree1/1(sync)
  ri_to_c0/1(c) -> out/1
  convert_2/1 -> ri_to_c0/2(im)
  convert_1/1 -> ri_to_c0/1(re)
  scale_2/1 -> convert_2/1
  adder_tree2/2(dout) -> scale_2/1
  mult2/2(c2) -> adder_tree2/3(din_2)
  mult2/1(c1) -> adder_tree2/2(din_1)
  tap_split_2/2(outport2) -> mult2/4(b2)
  tap_split_1/2(outport2) -> mult2/2(b1)
  sync_delay1/1 -> sync_out/1
  adder_tree1/1(sync_out) -> sync_delay1/1
  scale_1/1 -> convert_1/1
  adder_tree1/2(dout) -> scale_1/1
  mult1/2(c2) -> adder_tree1/3(din_2)
  mult1/1(c1) -> adder_tree1/2(din_1)
  tap_split_2/1(outport1) -> mult1/4(b2)
  tap_split_1/1(outport1) -> mult1/2(b1)
  delay_bram2/1(dout_1_1) -> tap_split_2/1(inport)
  pfb_coeff_gen/2(sync_out) -> sync_delay/1(In)
  sync/1 -> pfb_coeff_gen/2(sync)
  din/1 -> pfb_coeff_gen/1(din)

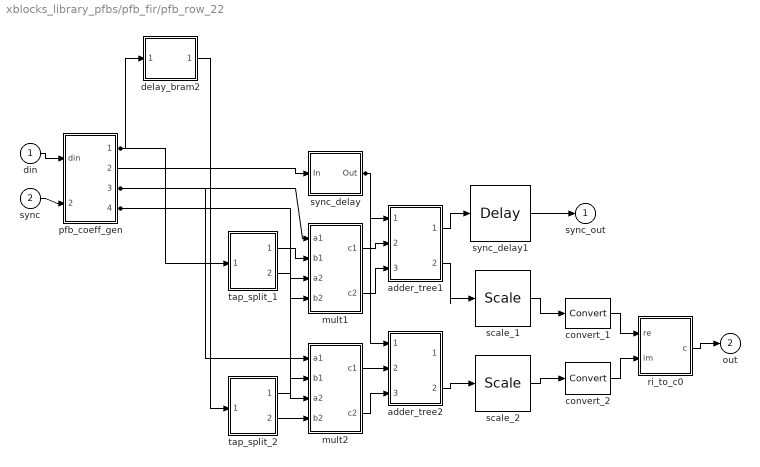
== system xblocks_library_pfbs/pfb_fir/pfb_row_22 ==
  din : Inport
  sync : Inport  Port=2
  adder_tree1 : Subsystem
  adder_tree2 : Subsystem
  convert_1 : xbsIndex_r4/Convert  gui_display_data_type=Fixed-point  arith_type="Signed  (2's comp)"  n_bits=18  bin_pt=17  float_type=Single  exp_bits=8  fraction_bits=24  quantization="Round  (unbiased: +/- Inf)"  overflow=Saturate  en=off  latency=2  dbl_ovrd=off  pipeline=on  block_type=convert
  convert_2 : xbsIndex_r4/Convert  gui_display_data_type=Fixed-point  arith_type="Signed  (2's comp)"  n_bits=18  bin_pt=17  float_type=Single  exp_bits=8  fraction_bits=24  quantization="Round  (unbiased: +/- Inf)"  overflow=Saturate  en=off  latency=2  dbl_ovrd=off  pipeline=on  block_type=convert
  delay_bram2 : Subsystem
  mult1 : Subsystem
  mult2 : Subsystem
  pfb_coeff_gen : Subsystem
      settings: AttributesFormatString=PFBSize=5, n_inputs=1, taps=2
  ri_to_c0 : Subsystem
  scale_1 : xbsIndex_r4/Scale  scale_factor=-2  dbl_ovrd=off  block_type=scale
  scale_2 : xbsIndex_r4/Scale  scale_factor=-2  dbl_ovrd=off  block_type=scale
  sync_delay : Subsystem
  sync_delay1 : xbsIndex_r4/Delay  rst=off  infoeditControl=Selection of Reset will increase slice count due to use of real FFs and instead of SRLs  en=off  latency=2  dbl_ovrd=off  reg_retiming=off  block_type=delay
  tap_split_1 : Subsystem
      settings: AttributesFormatString=Fix_8_7
  tap_split_2 : Subsystem
      settings: AttributesFormatString=Fix_8_7
  sync_out : Outport
  out : Outport  Port=2
  wires:
  pfb_coeff_gen/1(dout) -> tap_split_1/1(inport), delay_bram2/1(din_1_1)
  pfb_coeff_gen/3(coeffs1) -> mult2/1(a1), mult1/1(a1)
  pfb_coeff_gen/4(coeffs2) -> mult2/3(a2), mult1/3(a2)
  sync_delay/1(Out) -> adder_tree2/1(sync), adder_tree1/1(sync)
  ri_to_c0/1(c) -> out/1
  convert_2/1 -> ri_to_c0/2(im)
  convert_1/1 -> ri_to_c0/1(re)
  scale_2/1 -> convert_2/1
  adder_tree2/2(dout) -> scale_2/1
  mult2/2(c2) -> adder_tree2/3(din_2)
  mult2/1(c1) -> adder_tree2/2(din_1)
  tap_split_2/2(outport2) -> mult2/4(b2)
  tap_split_1/2(outport2) -> mult2/2(b1)
  sync_delay1/1 -> sync_out/1
  adder_tree1/1(sync_out) -> sync_delay1/1
  scale_1/1 -> convert_1/1
  adder_tree1/2(dout) -> scale_1/1
  mult1/2(c2) -> adder_tree1/3(din_2)
  mult1/1(c1) -> adder_tree1/2(din_1)
  tap_split_2/1(outport1) -> mult1/4(b2)
  tap_split_1/1(outport1) -> mult1/2(b1)
  delay_bram2/1(dout_1_1) -> tap_split_2/1(inport)
  pfb_coeff_gen/2(sync_out) -> sync_delay/1(In)
  sync/1 -> pfb_coeff_gen/2(sync)
  din/1 -> pfb_coeff_gen/1(din)
